simulink model "GS_model"  (R2018b)
settings: Solver=ode5  StartTime=0.0  StopTime=SimuStopTime  FixedStep=T_Simu  RelTol=1e-3
InitFcn:
  | Initial
undefined symbols (not defined in the file or in its folder): Aba10, Aba20, aeroCIP2006_S, aeroCIP2006_X, aeroCIP2006_Y, Agl0, Ass_kS, Ass_n1, Ass_n2, Ass_n3, Ass_n4, Ass_Noise, Ass_R, Ass_Resolution, Ass_TmOrder, AssA_Fix_Abs, AssB_Fix_Abs, AssC_Fix_Abs, AssD_Fix_Abs, AssE_Fix_Aps, AssF_Fix_Aps, C, c_max, c_min, Cd, CenterOfFigNX, CenterOfFigNY, CenterOfFigNZ, CenterOfFigP1, CenterOfFigP2, CenterOfFigPX, CenterOfFigPY, CenterOfFigPZ, Cmu, Crou, DEG2RAD, DiscIntNeverNeededParam, Eg_Dir, Eg_F, Eg_PrepareTime, Eg_r_L_L, Fw_Abf, Fw_Hmax, Fw_J, Fw_Spd0, Fw_Tmax, git_hash_BaseLine, git_hash_Project, Gnss_Noise_Pos, Gnss_Noise_Vel, Gnss_PropgationTime, GyroA_Fix_Abg, GyroA_Noise, GyroB_Fix_Abg, GyroB_Noise, GyroC_Fix_Abg, GyroC_Noise, GyroD_Fix_Abg, GyroD_Noise, h ... (+94)
libraries: simulink x308, sharedutil x46, aerolibutil x37, sharedtransform x31, vrlib x14, aerolibgravity2 x2
(part 3 of 20)

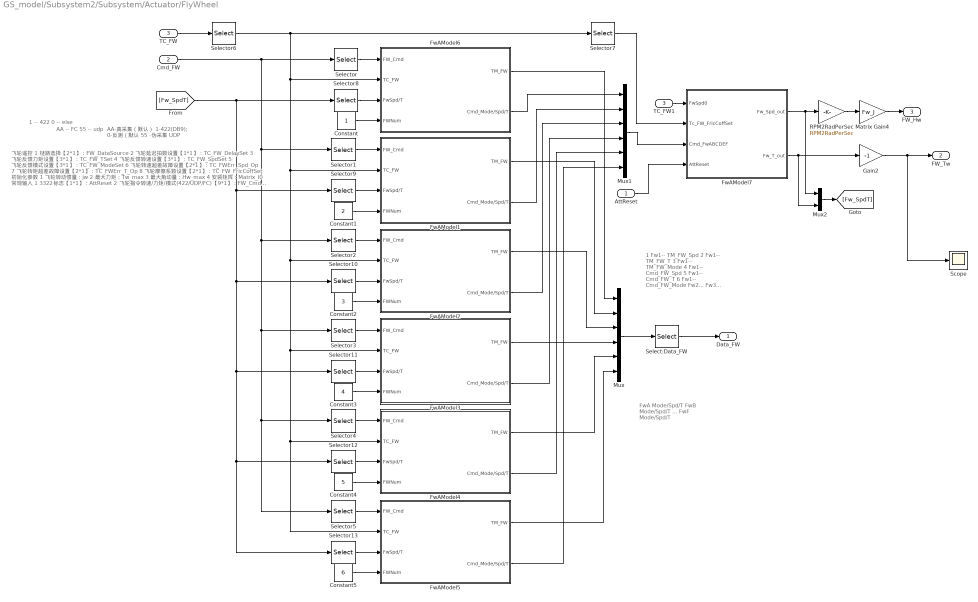
== system GS_model/Subsystem2/Subsystem/Actuator/FlyWheel ==
  note: FwA Mode/Spd/T
      | FwB Mode/Spd/T
      | ...
      | FwF Mode/Spd/T
  note: AA-真采集（默认）  1-422(DB9);
      |                                  0-反测（默认
      | 55 -伪采集                UDP
  note: 飞轮遥控
      | 1 链路选择【2*1】：FW_DataSource
      | 2 飞轮延迟拍数设置【1*1】：TC_FW_DelaySet
      | 3 飞轮反馈力矩设置【3*1】：TC_FW_TSet
      | 4 飞轮反馈转速设置【3*1】：TC_FW_SpdSet
      | 5 飞轮反馈模式设置【3*1】：TC_FW_ModeSet
      | 6 飞轮转速超差故障设置【2*1】：TC_FWErr_Spd_Op
      | 7 飞轮转矩超差故障设置【2*1】：TC_FWErr_T_Op
      | 8 飞轮摩擦系数设置【2*1】：TC_FW_FricCoffSet
      |
      | 初始化参数
      | 1 飞轮转动惯量：jw
      | 2 最大力矩：Tw_max
      | 3 最大角动量：Hw_max
      | 4 安装矩阵：Matrix_I0
      |
      | 常规输入
      | 1 3322标志【1*1】：AttReset
      | 2 飞轮指令转速/力矩/模式(422/UDP/FC)【9*1】：FW_Cmd
      |
      | 常规输出
      | 1 飞轮三轴力矩FW_Tw3
      | 2 飞轮三轴角动量：FW_Hw3
      |
      | 遥测输出
      | 1 飞轮反馈转速/力矩/模式【18*1】：Data_FW
  note: AA -- FC
      | 55 -- udp
  note: 1 -- 422
      | 0 -- else
  note: 1 Fw1-- TM_FW_Spd
      | 2 Fw1-- TM_FW_T
      | 3 Fw1-- TM_FW_Mode
      | 4 Fw1-- Cmd_FW_Spd
      | 5 Fw1-- Cmd_FW_T
      | 6 Fw1-- Cmd_FW_Mode
      |    Fw2...
      |    Fw3...
  AttReset : Inport
  Cmd_FW : Inport  Port=2
  TC_FW : Inport  Port=3
  Constant : Constant
  Constant1 : Constant  Value=2
  Constant2 : Constant  Value=3
  Constant3 : Constant  Value=4
  Constant4 : Constant  Value=5
  Constant5 : Constant  Value=6
  FwAModel1 : Subsystem
      mask Display: disp('FwAModel')
  FwAModel2 : Subsystem
      mask Display: disp('FwAModel')
  FwAModel3 : Subsystem
      mask Display: disp('FwAModel')
  FwAModel4 : Subsystem
      mask Display: disp('FwAModel')
  FwAModel5 : Subsystem
      mask Display: disp('FwAModel')
  FwAModel6 : Subsystem
      mask Display: disp('FwAModel')
  FwAModel7 : Subsystem
      mask Display: disp('FwModel')
  Gain2 : Gain  Gain=-1  SaturateOnIntegerOverflow=on  OutDataTypeStr=Inherit: Same as input  ParamDataTypeStr=Inherit: Same as input
  Matrix Gain4 : Gain  Gain=Fw_J  SaturateOnIntegerOverflow=on  OutDataTypeStr=Inherit: Same as input  ParamDataTypeStr=Inherit: Same as input
  Mux : Mux  Inputs=6
  Mux1 : Mux  Inputs=6
  Mux2 : Mux  Inputs=2
  RPM2RadPerSec : Gain  Gain=RPM2RadPerSec  SaturateOnIntegerOverflow=on  OutDataTypeStr=Inherit: Same as input  ParamDataTypeStr=Inherit: Same as input
  Scope : Scope
  Select:Data_FW : Selector  InputPortWidth=8*6  IndexOptions=Index vector (dialog)  Indices=[1:6 9:14 17:22 25:30 33:38 41:46]  OutputSizes=1
  Selector : Selector  InputPortWidth=18  IndexOptions=Index vector (dialog)  Indices=[1:3]  OutputSizes=1
  Selector1 : Selector  InputPortWidth=18  IndexOptions=Index vector (dialog)  Indices=[4:6]  OutputSizes=1
  Selector10 : Selector  InputPortWidth=12  IndexOptions=Index vector (dialog)  Indices=[3 9]  OutputSizes=1
  Selector11 : Selector  InputPortWidth=12  IndexOptions=Index vector (dialog)  Indices=[4 10]  OutputSizes=1
  Selector12 : Selector  InputPortWidth=12  IndexOptions=Index vector (dialog)  Indices=[5 11]  OutputSizes=1
  Selector13 : Selector  InputPortWidth=12  IndexOptions=Index vector (dialog)  Indices=[6 12]  OutputSizes=1
  Selector2 : Selector  InputPortWidth=18  IndexOptions=Index vector (dialog)  Indices=[7:9]  OutputSizes=1
  Selector3 : Selector  InputPortWidth=18  IndexOptions=Index vector (dialog)  Indices=[10:12]  OutputSizes=1
  Selector4 : Selector  InputPortWidth=18  IndexOptions=Index vector (dialog)  Indices=[13:15]  OutputSizes=1
  Selector5 : Selector  InputPortWidth=18  IndexOptions=Index vector (dialog)  Indices=[16:18]  OutputSizes=1
  Selector6 : Selector  InputPortWidth=23  IndexOptions=Index vector (dialog)  Indices=[3:17]  OutputSizes=1
  Selector7 : Selector  InputPortWidth=15  IndexOptions=Index vector (dialog)  Indices=15  OutputSizes=1
  Selector8 : Selector  InputPortWidth=12  IndexOptions=Index vector (dialog)  Indices=[1 7]  OutputSizes=1
  Selector9 : Selector  InputPortWidth=12  IndexOptions=Index vector (dialog)  Indices=[2 8]  OutputSizes=1
  TC_FW1 : InportShadow  Port=3
  Data_FW : Outport
  FW_Tw : Outport  Port=2
  FW_Hw : Outport  Port=3
  wires:
  Gain2/1 -> Scope/1, FW_Tw/1
  Matrix Gain4/1 -> FW_Hw/1
  Selector6/1 -> FwAModel5/2(TC_FW), FwAModel4/2(TC_FW), FwAModel3/2(TC_FW), FwAModel2/2(TC_FW), FwAModel1/2(TC_FW), FwAModel6/2(TC_FW), Selector7/1
  Selector5/1 -> FwAModel5/1(FW_Cmd)
  Selector4/1 -> FwAModel4/1(FW_Cmd)
  TC_FW/1 -> Selector6/1
  Cmd_FW/1 -> Selector5/1, Selector4/1, Selector3/1, Selector2/1, Selector1/1, Selector/1
  Select:Data_FW/1 -> Data_FW/1
  FwAModel7/1(Fw_Spd_out) -> Mux2/1, RPM2RadPerSec/1
  FwAModel5/1(TM_FW) -> Mux/6
  FwAModel4/1(TM_FW) -> Mux/5
  FwAModel3/1(TM_FW) -> Mux/4
  FwAModel2/1(TM_FW) -> Mux/3
  FwAModel1/1(TM_FW) -> Mux/2
  FwAModel6/1(TM_FW) -> Mux/1
  RPM2RadPerSec/1 -> Matrix Gain4/1
  FwAModel7/2(Fw_T_out) -> Mux2/2, Gain2/1
  Mux/1 -> Select:Data_FW/1
  Selector3/1 -> FwAModel3/1(FW_Cmd)
  Selector2/1 -> FwAModel2/1(FW_Cmd)
  Selector1/1 -> FwAModel1/1(FW_Cmd)
  Constant/1 -> FwAModel6/4(FWNum)
  Selector/1 -> FwAModel6/1(FW_Cmd)
  AttReset/1 -> FwAModel7/4(AttReset)
  Constant1/1 -> FwAModel1/4(FWNum)
  Constant2/1 -> FwAModel2/4(FWNum)
  Constant3/1 -> FwAModel3/4(FWNum)
  Constant4/1 -> FwAModel4/4(FWNum)
  Constant5/1 -> FwAModel5/4(FWNum)
  FwAModel6/2(Cmd_Mode/Spd/T) -> Mux1/1
  FwAModel1/2(Cmd_Mode/Spd/T) -> Mux1/2
  FwAModel2/2(Cmd_Mode/Spd/T) -> Mux1/3
  FwAModel3/2(Cmd_Mode/Spd/T) -> Mux1/4
  FwAModel4/2(Cmd_Mode/Spd/T) -> Mux1/5
  FwAModel5/2(Cmd_Mode/Spd/T) -> Mux1/6
  Selector7/1 -> FwAModel7/2(Tc_FW_FricCoffSet)
  Mux1/1 -> FwAModel7/3(Cmd_FwABCDEF)
  [Fw_SpdT] -> Selector8/1, Selector9/1, Selector10/1, Selector11/1, Selector12/1, Selector13/1
  Selector8/1 -> FwAModel6/3(FwSpd/T)
  Selector9/1 -> FwAModel1/3(FwSpd/T)
  Selector10/1 -> FwAModel2/3(FwSpd/T)
  Selector11/1 -> FwAModel3/3(FwSpd/T)
  Selector12/1 -> FwAModel4/3(FwSpd/T)
  Selector13/1 -> FwAModel5/3(FwSpd/T)
  Mux2/1 -> [Fw_SpdT]
  TC_FW1/1 -> FwAModel7/1(FwSpd0)

== system GS_model/Subsystem2/Subsystem/Actuator/Magnetorquer ==
  Tc_Mt : Inport
  Cmd_Mt : Inport  Port=2
  Mt_MathModel : Subsystem
  Mux : Mux  Inputs=2
  Data_Mt : Outport
  M_Mt : Outport  Port=2
  wires:
  Tc_Mt/1 -> Mt_MathModel/2(Tc_Mt)
  Cmd_Mt/1 -> Mt_MathModel/1(Cmd_Mt_Pro)
  Mt_MathModel/3(Tm_Mt) -> Mux/2
  Mt_MathModel/2(Cmd_Mt) -> Mux/1
  Mux/1 -> Data_Mt/1
  Mt_MathModel/1(M_Mt) -> M_Mt/1

== system GS_model/Subsystem2/Subsystem/Actuator/Motor ==
  Att_Reset : Inport
  Cmd_Motor : Inport  Port=2
  Tc_SADA : Inport  Port=3
  Tc_QV : Inport  Port=4
  UTC_1970 : Inport  Port=5
  Mux : Mux  Inputs=2
  QV : Subsystem
  Rate Transition{,1..2,4} (4 alike) : RateTransition  OutPortSampleTime=T_Simu
  SADA : Subsystem
  Selector1 : Selector  InputPortWidth=30  IndexOptions=Starting index (dialog)  Indices=1  OutputSizes=12
  Selector2 : Selector  InputPortWidth=30  IndexOptions=Starting index (dialog)  Indices=13  OutputSizes=8
  Selector3 : Selector  InputPortWidth=30  IndexOptions=Starting index (dialog)  Indices=21  OutputSizes=6
  Selector4 : Selector  InputPortWidth=30  IndexOptions=Starting index (dialog)  Indices=27  OutputSizes=4
  Motor_Agl/w/a : Outport
  Data_SADA : Outport  Port=2
  Data_QV : Outport  Port=3
  wires:
  Att_Reset/1 -> Rate Transition2/1
  Cmd_Motor/1 -> Selector3/1, Selector4/1, Selector2/1, Selector1/1
  Tc_SADA/1 -> Rate Transition/1
  SADA/1(Data_Motor_out) -> Data_SADA/1
  Rate Transition/1 -> SADA/1(TC_Motor_in)
  Rate Transition1/1 -> SADA/2(Cmd_Motor_in)
  Rate Transition2/1 -> QV/3(AttReset), SADA/3(AttReset)
  Selector1/1 -> Rate Transition1/1
  Selector2/1 -> QV/2(Cmd_Motor_in)
  Rate Transition4/1 -> QV/1(TC_Motor_in)
  Tc_QV/1 -> Rate Transition4/1
  QV/1(Data_Motor_out) -> Data_QV/1
  QV/2(SADA_Agl/w/a) -> Mux/2
  Selector4/1 -> QV/4(QVAgl_FC)
  Selector3/1 -> SADA/4(SADAAgl_FC)
  SADA/2(SADA_Agl/w/a) -> Mux/1
  Mux/1 -> Motor_Agl/w/a/1
  UTC_1970/1 -> QV/5(UTC_1970), SADA/5(UTC_1970)

== system GS_model/Subsystem2/Subsystem/PhysicsModel/DynModel ==
  note: % 输入：三轴外力（b系） 三轴外力矩（b系） 飞轮三轴角动量 飞轮三轴角动量微分
      | % 输入：a1角度/角速度/角加速度 p1角度/角速度/角加速度 附件1转序
      | % 输入：a2角度/角速度/角加速度 p2角度/角速度/角加速度 附件2转序
      | % 输入：上一拍微分方程输出值
      | % 输出：R(i系) Qib q   V(i系) wbi dq
  RV0 : Inport
  Orbit : Inport  Port=2
  Qio : Inport  Port=3
  Hw : Inport  Port=4
  Att0 : Inport  Port=5
  F(i) : Inport  Port=6
  Reset : Inport  Port=7
  AscDec : Inport  Port=8
  T(b) : Inport  Port=9
  Tc_MassPropertySet : Inport  Port=10
  Motor_Agl/w/a : Inport  Port=11
  AngularMomentumConservation : Subsystem
  Att：ECEF2VVLH : Subsystem
  Demux1 : Demux  Outputs=2
  Discrete Derivative : simulink/Discrete/Discrete Derivative  gainval=1.0  ICPrevScaledInput=0.0  OutMin=[]  OutMax=[]  OutDataType=fixdt(1, 16)  OutScaling=2^-10  DoSatur=off
  Display1 : Display
  EulerAngle_Inertial : Subsystem
  FlexDynModel : Subsystem
  Gain2 : Gain  Gain=RAD2DEG
  Hi : Scope  NumInputPorts=2
  Mux : Mux  Inputs=3
  Quaternion Norm : sharedutil/Quaternion Norm  aMode=aMode
      settings: SourceProductBaseCode=AE,PW,MT,VE,VP
  Quaternions to Rotation Angles : sharedtransform/Quaternions to Rotation Angles  rotationOrder=ZYX  aMode=aMode
      settings: SourceProductBaseCode=AE,PW,MT,VE,VP
  Scope : Scope
  Selector : Selector  InputPortWidth=3  IndexOptions=Index vector (dialog)  Indices=[3 2 1]  OutputSizes=1
  Selector2 : Selector  InputPortWidth=10  IndexOptions=Index vector (dialog)  Indices=[9]  OutputSizes=1
  Terminator : Terminator
  Terminator1 : Terminator
  Terminator2 : Terminator
  "wbi " : Scope
  Qib : Outport
  Qob : Outport  Port=2
  I : Outport  Port=3
  Cent : Outport  Port=4
  wbo : Outport  Port=5
  wbi : Outport  Port=6
  tag scope: Att_DLX=global, Euler_i=global, Euler_o=global, q_panel=global
  wires:
  Discrete Derivative/1 -> FlexDynModel/3(dHw_in)
  T(b)/1 -> FlexDynModel/4(T(b)_in)
  Att0/1 -> FlexDynModel/6(Att0_in)
  RV0/1 -> FlexDynModel/7(RV0_in)
  Motor_Agl/w/a/1 -> FlexDynModel/9(SADA_Agl/w/a_a/p_in)
  F(i)/1 -> FlexDynModel/8(F(i)_in)
  FlexDynModel/5(q_out) -> [q_panel]
  FlexDynModel/6(dq_out) -> Terminator2/1
  Orbit/1 -> Selector2/1
  Quaternions to Rotation Angles/1 -> Selector/1
  Demux1/1 -> EulerAngle_Inertial/1(Asc)
  EulerAngle_Inertial/1(EulerAngle_Inertial) -> [Euler_i]
  Demux1/2 -> EulerAngle_Inertial/2(Dec)
  AscDec/1 -> Demux1/1
  Gain2/1 -> "wbi "/1
  Reset/1 -> FlexDynModel/1(Reset_in)
  Hw/1 -> Discrete Derivative/1, AngularMomentumConservation/4(Hw_b), FlexDynModel/2(Hw_in)
  FlexDynModel/1(R_out) -> Terminator/1
  FlexDynModel/2(V_out) -> Terminator1/1
  AngularMomentumConservation/1(H_i) -> Hi/1
  [Spread] -> FlexDynModel/11(Spread_in)
  Selector2/1 -> Att：ECEF2VVLH/3(w00)
  Att：ECEF2VVLH/1(Qob) -> Qob/1, Quaternions to Rotation Angles/1
  Qio/1 -> FlexDynModel/5(Agl_Qio_in), Att：ECEF2VVLH/4(Qio)
  Tc_MassPropertySet/1 -> FlexDynModel/10(Tc_MassPropertySet_in)
  FlexDynModel/3(Agl_Qib_out) -> Att：ECEF2VVLH/1(Qib), AngularMomentumConservation/1(Qib), Quaternion Norm/1, EulerAngle_Inertial/3(Qib), Qib/1
  FlexDynModel/4(wbi_out) -> Att：ECEF2VVLH/2(wbi_b), AngularMomentumConservation/2(Wbi_b), Mux/3, Gain2/1, wbi/1
  FlexDynModel/7(I_out) -> AngularMomentumConservation/3(Ib), I/1
  FlexDynModel/8(Cent_out) -> Display1/1, Cent/1
  Selector/1 -> Mux/1, [Euler_o]
  Att：ECEF2VVLH/2(wbo_b) -> Mux/2, wbo/1
  Mux/1 -> [Att_DLX]
  Quaternion Norm/1 -> Scope/1
  AngularMomentumConservation/2(|H_i|) -> Hi/2

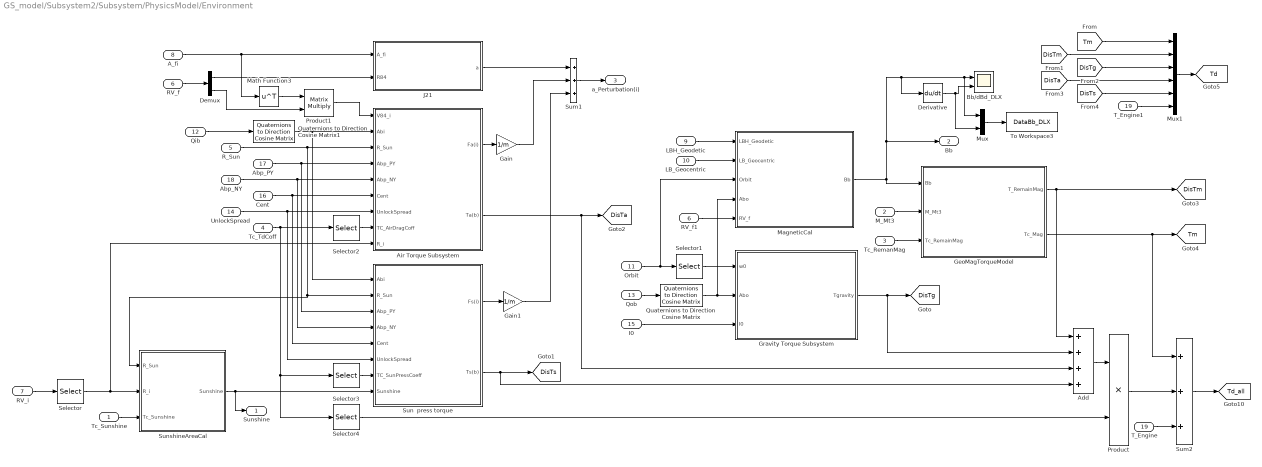
== system GS_model/Subsystem2/Subsystem/PhysicsModel/Environment ==
  Tc_Sunshine : Inport
  M_Mt3 : Inport  Port=2
  Tc_RemanMag : Inport  Port=3
  Tc_TdCoff : Inport  Port=4
  R_Sun : Inport  Port=5
  RV_f : Inport  Port=6
  RV_i : Inport  Port=7
  A_fi : Inport  Port=8
  LBH_Geodetic : Inport  Port=9
  LB_Geocentric : Inport  Port=10
  Orbit : Inport  Port=11
  Qib : Inport  Port=12
  Qob : Inport  Port=13
  UnlockSpread : Inport  Port=14
  I0 : Inport  Port=15
  Cent : Inport  Port=16
  Abp_PY : Inport  Port=17
  Abp_NY : Inport  Port=18
  T_Engine : Inport  Port=19
  Add : Sum  Inputs=++++
  Air Torque Subsystem : Subsystem
      mask Display: disp('AirDampModel')
  Bb/dBd_DLX : Scope  NumInputPorts=2
  Demux : Demux  Outputs=[3;3]
  Derivative : Derivative
  Gain : Gain  Gain=1/m
  Gain1 : Gain  Gain=1/m
  GeoMagTorqueModel : Subsystem
      mask Display: disp('GeoMagTorqueModel')
  Gravity Torque Subsystem : Subsystem
      mask Display: disp('GravityTorque')
  J21 : Subsystem
  MagneticCal : Subsystem
  Math Function3 : Math  Operator=transpose  SaturateOnIntegerOverflow=on
  Mux : Mux  Inputs=2
  Mux1 : Mux  Inputs=6
  Product : Product
  Product1 : Product  Multiplication=Matrix(*)
  Quaternions to Direction Cosine Matrix : sharedtransform/Quaternions to  Direction Cosine Matrix  aMode=aMode
      settings: SourceProductBaseCode=AE,PW,MT,VE,VP
  Quaternions to Direction Cosine Matrix1 : sharedtransform/Quaternions to  Direction Cosine Matrix  aMode=aMode
      settings: SourceProductBaseCode=AE,PW,MT,VE,VP
  RV_f1 : InportShadow  Port=6
  Selector : Selector  InputPortWidth=6  IndexOptions=Index vector (dialog)  Indices=[1 2 3]  OutputSizes=1
  Selector1 : Selector  InputPortWidth=10  IndexOptions=Index vector (dialog)  Indices=9  OutputSizes=1
  Selector2 : Selector  InputPortWidth=3  IndexOptions=Index vector (dialog)  Indices=1  OutputSizes=1
  Selector3 : Selector  InputPortWidth=3  IndexOptions=Index vector (dialog)  Indices=2  OutputSizes=1
  Selector4 : Selector  InputPortWidth=3  IndexOptions=Index vector (dialog)  Indices=3  OutputSizes=1
  Sum1 : Sum  Inputs=+++
  Sum2 : Sum  Inputs=3
  Sun  press torque : Subsystem
      mask Display: disp('SunPressModel')
  SunshineAreaCal : Subsystem
  T_Engine1 : InportShadow  Port=19
  To Workspace3 : ToWorkspace  VariableName=DataBb_DLX  SampleTime=-1
  Sunshine : Outport
  Bb : Outport  Port=2
  a_Perturbation(i) : Outport  Port=3
  tag scope: DisTa=global, DisTg=global, DisTm=global, DisTs=global, Td=global, Td_all=global, Tm=global
  wires:
  RV_f/1 -> Demux/1
  Demux/1 -> J21/2(R84)
  Math Function3/1 -> Product1/1
  A_fi/1 -> Math Function3/1, J21/1(A_fi)
  M_Mt3/1 -> GeoMagTorqueModel/2(M_Mt3)
  Demux/2 -> Product1/2
  Product1/1 -> Air Torque Subsystem/1(V84_i)
  Qib/1 -> Quaternions to Direction Cosine Matrix1/1
  R_Sun/1 -> SunshineAreaCal/1(R_Sun), Sun  press torque/2(R_Sun), Air Torque Subsystem/3(R_Sun)
  Abp_PY/1 -> Sun  press torque/3(Abp_PY), Air Torque Subsystem/4(Abp_PY)
  Abp_NY/1 -> Sun  press torque/4(Abp_NY), Air Torque Subsystem/5(Abp_NY)
  Cent/1 -> Sun  press torque/5(Cent), Air Torque Subsystem/6(Cent)
  UnlockSpread/1 -> Sun  press torque/6(UnlockSpread), Air Torque Subsystem/7(UnlockSpread)
  Tc_TdCoff/1 -> Selector4/1, Selector3/1, Selector2/1
  RV_i/1 -> Selector/1
  Selector/1 -> SunshineAreaCal/2(R_i), Air Torque Subsystem/9(R_i)
  Sum1/1 -> a_Perturbation(i)/1
  Air Torque Subsystem/1(Fa(i)) -> Gain/1
  I0/1 -> Gravity Torque Subsystem/3(I0)
  Qob/1 -> Quaternions to Direction Cosine Matrix/1
  Selector1/1 -> Gravity Torque Subsystem/1(w0)
  Orbit/1 -> Selector1/1, MagneticCal/3(Orbit)
  Quaternions to Direction Cosine Matrix/1 -> MagneticCal/4(Abo), Gravity Torque Subsystem/2(Abo)
  Selector2/1 -> Air Torque Subsystem/8(TC_AirDragCoff)
  Selector3/1 -> Sun  press torque/7(TC_SunPressCoeff)
  SunshineAreaCal/1(Sunshine) -> Sun  press torque/8(Sunshine), Sunshine/1
  Sun  press torque/1(Fs(i)) -> Gain1/1
  Gain1/1 -> Sum1/3
  LB_Geocentric/1 -> MagneticCal/2(LB_Geocentric)
  LBH_Geodetic/1 -> MagneticCal/1(LBH_Geodetic)
  MagneticCal/1(Bb) -> GeoMagTorqueModel/1(Bb), Derivative/1, Mux/1, Bb/dBd_DLX/1, Bb/1
  Tc_RemanMag/1 -> GeoMagTorqueModel/3(Tc_RemainMag)
  Gravity Torque Subsystem/1(Tgravity) -> Add/2, [DisTg]
  GeoMagTorqueModel/2(Tc_Mag) -> Sum2/1, [Tm]
  Quaternions to Direction Cosine Matrix1/1 -> Sun  press torque/1(Abi), Air Torque Subsystem/2(Abi)
  Sum2/1 -> [Td_all]
  Tc_Sunshine/1 -> SunshineAreaCal/3(Tc_Sunshine)
  Sun  press torque/2(Ts(b)) -> [DisTs], Add/4
  Air Torque Subsystem/2(Ta(b)) -> Add/3, [DisTa]
  GeoMagTorqueModel/1(T_RemainMag) -> Add/1, [DisTm]
  J21/1(a) -> Sum1/1
  Gain/1 -> Sum1/2
  Derivative/1 -> Mux/2, Bb/dBd_DLX/2
  Mux/1 -> To Workspace3/1
  Add/1 -> Product/1
  Selector4/1 -> Product/2
  Product/1 -> Sum2/2
  T_Engine/1 -> Sum2/3
  Mux1/1 -> [Td]
  [DisTm] -> Mux1/2
  [Tm] -> Mux1/1
  [DisTg] -> Mux1/3
  [DisTa] -> Mux1/4
  [DisTs] -> Mux1/5
  T_Engine1/1 -> Mux1/6
  RV_f1/1 -> MagneticCal/5(RV_f)

== system GS_model/Subsystem2/Subsystem/PhysicsModel/Environment1 ==
  JDC_2000 : Inport
  Constant : Constant  Value=[0;0;0]
  Constant1 : Constant  Value=[0;0]
  MATLAB Function : MATLAB Function  TreatAsAtomicUnit=on
  AscDec_Sun : Outport
  R_Moon : Outport  Port=2
  AscDec_Moon : Outport  Port=3
  R_Sun : Outport  Port=4
  wires:
  JDC_2000/1 -> MATLAB Function/1(JDC_2000)
  MATLAB Function/2(AscDec_Sun) -> AscDec_Sun/1
  Constant/1 -> R_Moon/1
  Constant1/1 -> AscDec_Moon/1
  MATLAB Function/1(R_Sun) -> R_Sun/1

== system GS_model/Subsystem2/Subsystem/PhysicsModel/Orbit ==
  UTC_1970 : Inport
  Tc_Reset : Inport  Port=2
  Tc_Orbit : Inport  Port=3
  F_Engine(b) : Inport  Port=4
  Qib : Inport  Port=5
  a_Perturbation : Inport  Port=6
  Compute osculating elements : Subsystem
  Engine : Subsystem
  Fcn : Fcn  Expr=u(5)+u(6)
  Gain : Gain  Gain=180/pi
  MATLAB Function : MATLAB Function  TreatAsAtomicUnit=on
  MATLAB Function1 : MATLAB Function  TreatAsAtomicUnit=on
  Mux : Mux  Inputs=2
  Mux1 : Mux  Inputs=2
  Mux2 : Mux  Inputs=3
  Mux3 : Mux  Inputs=3
  Qob 2 Qib : Subsystem
  RV_i2RV_f : Subsystem
  Selector : Selector  InputPortWidth=2  IndexOptions=Index vector (dialog)  Indices=1  OutputSizes=1
  Subsystem : Subsystem
  Subsystem1 : Subsystem
  u : Scope
  RV_f : Outport
  RV_i : Outport  Port=2
  Afi : Outport  Port=3
  LBH_Geodetic : Outport  Port=4
  LBH_Geocentic : Outport  Port=5
  Orbit : Outport  Port=6
  Qio : Outport  Port=7
  RV0 : Outport  Port=8
  tag scope: LBH=global, Orbit=global
  wires:
  a_Perturbation/1 -> Subsystem/3(a_Perturbation)
  Subsystem/2(V_i) -> RV_i2RV_f/2(V_i), Mux/2, Compute osculating elements/2(v_xyz)
  Subsystem/1(R_i) -> RV_i2RV_f/1(R_i), Mux/1, Compute osculating elements/1(r_xyz)  "不对"
  Mux/1 -> RV_i/1
  Compute osculating elements/1(OrbitElement) -> Fcn/1, [Orbit], Qob 2 Qib/1(OrbitElement), Orbit/1
  UTC_1970/1 -> Subsystem1/1(UTC_1970)
  RV_i2RV_f/1(R_f) -> Mux1/1, MATLAB Function/1(R_84)
  Subsystem1/1(Afi) -> Afi/1, RV_i2RV_f/3(Afi)
  RV_i2RV_f/2(V_f) -> Mux1/2
  Mux1/1 -> RV_f/1
  MATLAB Function/1(L_Geodetic) -> Mux2/1
  MATLAB Function/2(B_Geodetic) -> Mux2/2
  MATLAB Function/3(H_Geodetic) -> Mux2/3
  MATLAB Function/4(L_Geocentric) -> Mux3/1
  MATLAB Function/5(B_Geocentric) -> Mux3/2
  Selector/1 -> Subsystem/1(Tc_Orbit_Reset)
  Tc_Reset/1 -> Selector/1
  Qob 2 Qib/1(Qio) -> Qio/1
  Tc_Orbit/1 -> MATLAB Function1/1(Orbit)
  MATLAB Function1/1(RV_i) -> RV0/1, Subsystem/2(RV0)
  Mux2/1 -> LBH_Geodetic/1, [LBH]  "地理"
  Mux3/1 -> LBH_Geocentic/1  "地心"
  Fcn/1 -> Gain/1
  Gain/1 -> u/1
  Qib/1 -> Engine/2(Qib)
  F_Engine(b)/1 -> Engine/1(F_Engine(b))
  Engine/1(F_Engine(i)) -> Subsystem/4(F_EP)
  MATLAB Function/6(H_Geocentric) -> Mux3/3

== system GS_model/Subsystem2/Subsystem/PhysicsModel/Subsystem3 ==
  M_Mt : Inport
  H_Fw : Inport  Port=2
  T_Fw : Inport  Port=3
  Agl/w/a_SADA : Inport  Port=4
  Gain : Gain  Gain=Mt_Abm  Multiplication=Matrix(K*u)
  Gain1 : Gain  Gain=Fw_Abf  Multiplication=Matrix(K*u)
  Gain2 : Gain  Gain=Fw_Abf  Multiplication=Matrix(K*u)
  Selector1 : Selector  InputPortWidth=30  IndexOptions=Index vector (dialog)  Indices=1:12  OutputSizes=1
  Subsystem1 : Subsystem
  Terminator : Terminator
  Terminator1 : Terminator
  Abp_PY : Outport
  Abp_NY : Outport  Port=2
  M_Dyn : Outport  Port=3
  H_Dyn : Outport  Port=4
  tag scope: T_Fw3=global
  wires:
  Gain2/1 -> H_Dyn/1
  Gain/1 -> M_Dyn/1
  M_Mt/1 -> Gain/1
  T_Fw/1 -> Gain1/1
  H_Fw/1 -> Gain2/1
  Gain1/1 -> [T_Fw3]
  Subsystem1/1(Abp1) -> Abp_PY/1
  Subsystem1/2(Aba1) -> Terminator/1
  Subsystem1/3(Abp2) -> Abp_NY/1
  Subsystem1/4(Aba2) -> Terminator1/1
  Agl/w/a_SADA/1 -> Selector1/1
  Selector1/1 -> Subsystem1/1(Agl/w/a_SADA)

== system GS_model/Subsystem2/Subsystem/PhysicsModel/Time ==
  UTC0_1970 : Inport
  Reset : Inport  Port=2
  Clock : Clock
  Constant : Constant  Value=UTC_1970to2000
  Constant2 : Constant  Value=T_LeapSec
  Gain : Gain  Gain=1/K_Day2Sec
  Gain1 : Gain  Gain=1/K_Century2Day
  Selector : Selector  InputPortWidth=2  IndexOptions=Index vector (dialog)  Indices=1  OutputSizes=1
  Subsystem : Subsystem
  Sum : Sum  Inputs=|+-
  Sum1 : Sum  Inputs=|++
  Sum2 : Sum  Inputs=-+|
  Sum3 : Sum  Inputs=|++
  JDC_2000 : Outport
  TAI_1970 : Outport  Port=2
  UTC_1970 : Outport  Port=3
  wires:
  Sum/1 -> Gain/1
  Constant/1 -> Sum/2
  Gain/1 -> Gain1/1
  Gain1/1 -> JDC_2000/1
  UTC0_1970/1 -> Sum3/2
  Reset/1 -> Selector/1
  Constant2/1 -> Sum1/1
  Sum3/1 -> Sum1/2, UTC_1970/1, Sum/1
  Sum1/1 -> TAI_1970/1
  Selector/1 -> Subsystem/Trigger
  Clock/1 -> Sum2/2, Subsystem/1(In1)
  Subsystem/1(Out1) -> Sum2/1
  Sum2/1 -> Sum3/1

== system GS_model/Subsystem2/Subsystem/Sensor/Ass ==
  note: 太敏遥控
      | 1 电池片设置【6*1】：TC_AssGNDSet
      | 2 不变故障【2*1】：TC_AssErr_Constant
      | 3 野值故障【2*1】：TC_AssErr_WildValue
      | 4 跳变故障【4*1】：TC_AssErr_Jump
      | 5 波动故障【3*1】：TC_AssErr_Wave
      |
      | 初始化参数
      | 1 安装矩阵【3*3】：AssA/B/C/D_Fix_Abs (Body)
      | 2 安装矩阵【3*3】：AssE_Fix_Aps (PY)
      | 3 安装矩阵【3*3】：AssF_Fix_Aps (NY)
      | 4 太敏电阻【1*1】：R_Ass
      |
      | 常规输入
      | 1 光照标志【1*1】：Sunshine
      | 2 本体系太阳矢量【3*1】：Sun_b
      | 3 正Y帆板转移矩阵【3*3】：Abp_PY
      | 4 负Y帆板转移矩阵【3*3】：Abp_NY
      |
      | 输出
      | 1 太敏电池片电流【24*1】：Data_Ass
  Sun_b : Inport
  Sunshine : Inport  Port=2
  TC_Ass : Inport  Port=3
  Abp_PY : Inport  Port=4
  Abp_NY : Inport  Port=5
  BodyAss(A&B&C&D)Model : Subsystem
      mask Display: disp('BodyAss(A&B&C&D)Model')
  Mux : Mux  Inputs=2
  SolarPanelAss(E&F)Model : Subsystem
      mask Display: disp('SolarPanelAss(E&F)Model');
  Data_Ass : Outport
  wires:
  Sunshine/1 -> SolarPanelAss(E&F)Model/1(Sunshine), BodyAss(A&B&C&D)Model/1(Sunshine)
  Sun_b/1 -> SolarPanelAss(E&F)Model/2(Sun_b), BodyAss(A&B&C&D)Model/2(Sun_b)
  TC_Ass/1 -> SolarPanelAss(E&F)Model/3(TC_Ass), BodyAss(A&B&C&D)Model/3(TC_Ass)
  BodyAss(A&B&C&D)Model/1(TM_Data_AssA&B&C&D) -> Mux/1
  Abp_PY/1 -> SolarPanelAss(E&F)Model/4(Abp_PY)
  Abp_NY/1 -> SolarPanelAss(E&F)Model/5(Abp_NY)
  SolarPanelAss(E&F)Model/1(TM_Data_AssE&F) -> Mux/2
  Mux/1 -> Data_Ass/1

== system GS_model/Subsystem2/Subsystem/Sensor/GNSS ==
  note: GNSS遥控
      | 1 位置设置【4*1】：TC_GNSS_GNDSet_Pos
      | 2 速度设置【4*1】：TC_GNSS_GNDSet_Spd
      | 3 位置不变故障【1*1】：TC_GNSSErr_PosConstant
      | 4 速度不变故障【1*1】：TC_GNSSErr_SpdConstant
      | 5 位置野值故障【1*1】：TC_GNSSErr_PosWildValue
      | 6 速度野值故障【1*1】：TC_GNSSErr_SpdWildValue
      | 7 外推时间【1*1】：TC_GNSS_T
      |
      | 初始化参数
      | 无
      |
      | 常规输入
      | 1 UTC1970【1*1】
      | 2 JDC2000【1*1】
      | 3 RV_J2000【6*1】
      |
      | 输出
      | GNSS时间/位置/速度/定位位置/定位速度【13*1】
  RV_f : Inport
  TC_GNSS : Inport  Port=2
  TAI1970 : Inport  Port=3
  UTC_1970 : Inport  Port=4
  Demux : Demux  Outputs=[3;3]
  Demux1 : Demux  Outputs=2
  Enabled Subsystem : Subsystem  TreatAsAtomicUnit=on
  GNSSErrModel : Subsystem
      mask Display: disp('GNSSErrModel')
  GNSS_IntegerSecond_Judge : Subsystem
  Gnss_Noise_Pos : RandomNumber  Mean=[0;0;0]  Variance=(Gnss_Noise_Pos/3).^2  Seed=[1;2;3]  SampleTime=T_Simu
  Gnss_Noise_Vel : RandomNumber  Mean=[0;0;0]  Variance=(Gnss_Noise_Vel/3).^2  Seed=[4;5;6]  SampleTime=T_Simu
  Mux : Mux  Inputs=5
  Mux1 : Mux  Inputs=2
  Mux2 : Mux  Inputs=2
  Mux3 : Mux  Inputs=2
  Orbit : Subsystem
      mask Display: disp('GNSS Propagation')
  Orbit1 : Subsystem
      mask Display: disp('GNSS Propagation')
  Sum : Sum  Inputs=|++
  Sum1 : Sum  Inputs=|++
  Sum2 : Sum  Inputs=|++
  Data_GNSS : Outport
  wires:
  Demux/1 -> GNSSErrModel/2(R_84)
  Demux/2 -> GNSSErrModel/3(V_84)
  GNSS_IntegerSecond_Judge/1(Boolean) -> Enabled Subsystem/Trigger
  TAI1970/1 -> Mux/1, GNSS_IntegerSecond_Judge/1(TAI1970)
  GNSSErrModel/1(TM_R_84) -> Mux/2
  GNSSErrModel/2(TM_V_84) -> Mux/3
  Mux/1 -> Enabled Subsystem/1(In1)
  Enabled Subsystem/1(Out1) -> Data_GNSS/1
  UTC_1970/1 -> Orbit1/2(UTC_1970), Orbit/2(UTC_1970)
  TC_GNSS/1 -> GNSSErrModel/1(TC_GNSS)
  Gnss_Noise_Vel/1 -> Mux1/2
  Gnss_Noise_Pos/1 -> Mux1/1
  RV_f/1 -> Sum/1
  Sum/1 -> Demux/1
  Demux1/1 -> Orbit/1("\tTC_GNSS_PropagationTime")
  Demux1/2 -> Orbit1/1("\tTC_GNSS_PropagationTime")
  Orbit1/1(R_f) -> Mux3/1
  Orbit1/2(V_f) -> Mux3/2
  Orbit/1(R_f) -> Mux2/1
  Orbit/2(V_f) -> Mux2/2
  Mux2/1 -> Sum1/1
  Mux3/1 -> Sum2/1
  Sum1/1 -> Mux/4
  Sum2/1 -> Mux/5
  GNSSErrModel/3(TC_GNSS_PropagationTime) -> Demux1/1
  Mux1/1 -> Sum1/2, Sum2/2, Sum/2

== system GS_model/Subsystem2/Subsystem/Sensor/Gyro ==
  note: 陀螺遥控
      | 1 TC_GyroGNDSet
      | 2 TC_GyroErr_Constant
      | 3 TC_GyroErr_WildValue
      | 4 TC_GyroErr_Jump
      | 5 TC_GyroErr_Wave
      | 6 TC_GyroDriftSet
      |
      | 初始化参数
      | 1   GyroA_Fix
      | 2   GyroB_Fix
      | 3   GyroC_Fix
      | 4   GyroD_Fix
      | 5   GyroA_Drift
      | 6   GyroB_Drift
      | 7   GyroC_Drift
      | 8   GyroD_Drift
      | 9   GyroA_Noise
      | 10 GyroB_Noise
      | 11 GyroC_Noise
      | 12 GyroD_Noise
      |
      | 常规输入
      | 1 Wbi
      |
      |
      | 输出
      | 1 Wgi_GyroA
      | 2 Wgi_GyroB
      | 3 Wgi_GyroC
      | 4 Wgi_GyroD
  Wbi_b : Inport
  Tc_Gyro : Inport  Port=2
  Constant : Constant
  Constant1 : Constant  Value=GyroA_Fix_Abg
  Constant10 : Constant  Value=GyroD_Fix_Abg
  Constant3 : Constant  Value=2
  Constant4 : Constant  Value=GyroB_Fix_Abg
  Constant6 : Constant  Value=3
  Constant7 : Constant  Value=GyroC_Fix_Abg
  Constant9 : Constant  Value=4
  GyroAModel : Subsystem
  GyroA_Noise : RandomNumber  Mean=[0;0;0]  Variance=(GyroA_Noise/180*pi/3).^2  Seed=[1;2;3]  SampleTime=T_Simu
  GyroBModel : Subsystem
  GyroB_Noise : RandomNumber  Mean=[0;0;0]  Variance=(GyroB_Noise/180*pi/3).^2  Seed=[1;2;3]+3  SampleTime=T_Simu
  GyroCModel : Subsystem
  GyroC_Noise : RandomNumber  Mean=[0;0;0]  Variance=(GyroC_Noise/180*pi/3).^2  Seed=[1;2;3]+6  SampleTime=T_Simu
  GyroDModel : Subsystem
  GyroD_Noise : RandomNumber  Mean=[0;0;0]  Variance=(GyroD_Noise/180*pi/3).^2  Seed=[1;2;3]+9  SampleTime=T_Simu
  Mux : Mux
  Data_Gyro : Outport
  wires:
  Wbi_b/1 -> GyroCModel/1(Wbi_b), GyroDModel/1(Wbi_b), GyroBModel/1(Wbi_b), GyroAModel/1(Wbi_b)
  Tc_Gyro/1 -> GyroAModel/4(TC_Gyro), GyroDModel/4(TC_Gyro), GyroCModel/4(TC_Gyro), GyroBModel/4(TC_Gyro)
  Constant1/1 -> GyroAModel/2(Gyro_Fix_Abg)
  GyroA_Noise/1 -> GyroAModel/3(Gyro_Noise)
  Mux/1 -> Data_Gyro/1
  GyroAModel/1(TM_Gyro_Wgi) -> Mux/1
  Constant/1 -> GyroAModel/5(Gyro_Num)
  GyroBModel/1(TM_Gyro_Wgi) -> Mux/2
  GyroCModel/1(TM_Gyro_Wgi) -> Mux/3
  GyroDModel/1(TM_Gyro_Wgi) -> Mux/4
  Constant4/1 -> GyroBModel/2(Gyro_Fix_Abg)
  GyroB_Noise/1 -> GyroBModel/3(Gyro_Noise)
  Constant3/1 -> GyroBModel/5(Gyro_Num)
  Constant7/1 -> GyroCModel/2(Gyro_Fix_Abg)
  GyroC_Noise/1 -> GyroCModel/3(Gyro_Noise)
  Constant6/1 -> GyroCModel/5(Gyro_Num)
  Constant10/1 -> GyroDModel/2(Gyro_Fix_Abg)
  GyroD_Noise/1 -> GyroDModel/3(Gyro_Noise)
  Constant9/1 -> GyroDModel/5(Gyro_Num)

== system GS_model/Subsystem2/Subsystem/Sensor/Magnetometer ==
  note: 磁强计遥控
      | 1 TC_MmGNDSet
      | 2 TC_MmErr_Constant
      | 3 TC_MmErr_WildValue
      | 4 TC_MmErr_Jump
      | 5 TC_MmErr_Wave
      |
      | 初始化参数
      | 1   MmA_Fix_Abm
      | 2   MmB_Fix_Abm
      | 3   MmC_Fix_Abm
      | 4   MmD_Fix_Abm
      | 5   MmA_MtInflunce_Coff
      | 6   MmB_MtInflunce_Coff
      | 7   MmC_MtInflunce_Coff
      | 8   MmD_MtInflunce_Coff
      | 9   Mt_MaxCurrent_Coff
      | 10 MmA_Noise
      | 11 MmB_Noise
      | 12 MmC_Noise
      | 13 MmD_Noise
      |
      | 常规输入
      | 1 Bb
      | 2 M_Mt
      |
      |
      | 输出
      | 1 MmA_MagneticIntensity
      | 2 MmB_MagneticIntensity
      | 3 MmC_MagneticIntensity
      | 4 MmD_MagneticIntensity
  Bb : Inport
  M_Mt : Inport  Port=2
  Tc_Mm : Inport  Port=3
  Constant11 : Constant  Value=MmB_Fix_Abm
  Constant12 : Constant  Value=MmB_MtInflunce_Coff
  Constant13 : Constant  Value=2
  Constant14 : Constant  Value=MmC_Fix_Abm
  Constant15 : Constant  Value=MmC_MtInflunce_Coff
  Constant16 : Constant  Value=3
  Constant17 : Constant  Value=MmD_Fix_Abm
  Constant18 : Constant  Value=MmD_MtInflunce_Coff
  Constant19 : Constant  Value=4
  Constant2 : Constant  Value=MmA_Fix_Abm
  Constant5 : Constant  Value=MmA_MtInflunce_Coff
  Constant8 : Constant
  Gain : Gain
  MmA_Noise : RandomNumber  Mean=[0;0;0]  Variance=(MmA_Noise/3).^2  Seed=[1;2;3]  SampleTime=T_Simu
  MmB_Noise : RandomNumber  Mean=[0;0;0]  Variance=(MmB_Noise/3).^2  Seed=[1;2;3]+3  SampleTime=T_Simu
  MmC_Noise : RandomNumber  Mean=[0;0;0]  Variance=(MmC_Noise/3).^2  Seed=[1;2;3]+6  SampleTime=T_Simu
  MmD_Noise : RandomNumber  Mean=[0;0;0]  Variance=(MmD_Noise/3).^2  Seed=[1;2;3]+9  SampleTime=T_Simu
  MmModel1 : Subsystem
  MmModel2 : Subsystem
  MmModel3 : Subsystem
  MmModel4 : Subsystem
  Mux1 : Mux
  Data_Mm : Outport
  wires:
  Constant2/1 -> MmModel1/3(Mm_Fix_Abm)
  Constant5/1 -> MmModel1/4(Mm_MtInflunce_Coff)
  MmA_Noise/1 -> MmModel1/5(Mm_Noise)
  Constant8/1 -> MmModel1/7(Mm_Num)
  Constant11/1 -> MmModel2/3(Mm_Fix_Abm)
  Constant12/1 -> MmModel2/4(Mm_MtInflunce_Coff)
  Constant13/1 -> MmModel2/7(Mm_Num)
  MmB_Noise/1 -> MmModel2/5(Mm_Noise)
  Constant14/1 -> MmModel3/3(Mm_Fix_Abm)
  Constant15/1 -> MmModel3/4(Mm_MtInflunce_Coff)
  Constant16/1 -> MmModel3/7(Mm_Num)
  MmC_Noise/1 -> MmModel3/5(Mm_Noise)
  Constant17/1 -> MmModel4/3(Mm_Fix_Abm)
  Constant18/1 -> MmModel4/4(Mm_MtInflunce_Coff)
  Tc_Mm/1 -> MmModel2/6(TC_Mm), MmModel4/6(TC_Mm), MmModel3/6(TC_Mm), MmModel1/6(TC_Mm)
  Constant19/1 -> MmModel4/7(Mm_Num)
  MmD_Noise/1 -> MmModel4/5(Mm_Noise)
  MmModel1/1(TM_Mm) -> Mux1/1
  MmModel2/1(TM_Mm) -> Mux1/2
  MmModel3/1(TM_Mm) -> Mux1/3
  MmModel4/1(TM_Mm) -> Mux1/4
  Mux1/1 -> Data_Mm/1
  M_Mt/1 -> MmModel2/2(M_Mt), MmModel4/2(M_Mt), MmModel3/2(M_Mt), MmModel1/2(M_Mt)
  Bb/1 -> Gain/1
  Gain/1 -> MmModel2/1(Bb), MmModel4/1(Bb), MmModel3/1(Bb), MmModel1/1(Bb)

== system GS_model/Subsystem2/Subsystem/Sensor/StA&B&C&DModel1 ==
  note: 星敏遥控
      | 1 TC_StFixErr
      | 2 TC_StNoiseCoff
      | 3 TC_StGNDSet
      | 4 TC_StErr_Constant
      | 5 TC_StErr_WildValue
      | 6 TC_StErr_Jump
      | 7 TC_StErr_Wave
      |
      | 初始化参数
      | 1 Qbs_StAFix
      | 2 Qbs_StBFix
      | 3 Qbs_StCFix
      | 4 Qbs_StDFix
      | 5 StANoise
      | 6 StBNoise
      | 7 StCNoise
      | 8 StDNoise
      |
      | 常规输入
      | 1 Qib
      | 2 UTC_1970
      |
      | 输出
      | 1 StA_Time/Qis_StA/W_StA
      | 2 StB_Time/Qis_StB/W_StB
      | 3 StC_Time/Qis_StC/W_StC
      | 4 StD_Time/Qis_StD/W_StD
  Qib : Inport
  Sun_b : Inport  Port=2
  Sunshine : Inport  Port=3
  TC_St : Inport  Port=4
  UTC_1970 : Inport  Port=5
  Qob : Inport  Port=6
  Constant : Constant  Value=StA_Fix_Qsb
  Constant1 : Constant
  Constant10 : Constant  Value=StC_Fix_Qsb
  Constant11 : Constant  Value=StD_Fix_Qsb
  Constant2 : Constant  Value=2
  Constant3 : Constant  Value=3
  Constant4 : Constant  Value=4
  Constant5 : Constant  Value=St_SEA
  Constant6 : Constant  Value=St_EEA
  Constant9 : Constant  Value=StB_Fix_Qsb
  Mux : Mux  Inputs=8
  Mux1 : Mux  Inputs=2
  Selector1 : Selector  InputPortWidth=4  IndexOptions=Index vector (dialog)  Indices=1  OutputSizes=1
  Selector2 : Selector  InputPortWidth=4  IndexOptions=Index vector (dialog)  Indices=1  OutputSizes=1
  Selector3 : Selector  InputPortWidth=4  IndexOptions=Index vector (dialog)  Indices=2  OutputSizes=1
  Selector4 : Selector  InputPortWidth=4  IndexOptions=Index vector (dialog)  Indices=2  OutputSizes=1
  Selector5 : Selector  InputPortWidth=4  IndexOptions=Index vector (dialog)  Indices=3  OutputSizes=1
  Selector6 : Selector  InputPortWidth=4  IndexOptions=Index vector (dialog)  Indices=3  OutputSizes=1
  Selector7 : Selector  InputPortWidth=4  IndexOptions=Index vector (dialog)  Indices=4  OutputSizes=1
  Selector8 : Selector  InputPortWidth=4  IndexOptions=Index vector (dialog)  Indices=4  OutputSizes=1
  StAMathModel : Subsystem
      mask Display: disp('StAModel');
  StAMathModel1 : Subsystem
      mask Display: disp('StAModel');
  StAMathModel2 : Subsystem
      mask Display: disp('StAModel');
  StAMathModel3 : Subsystem
      mask Display: disp('StAModel');
  StANoise : RandomNumber  Mean=[0;0;0]  Variance=(StANoise*pi/180/3600/3).^2  Seed=[1;2;3]  SampleTime=T_Simu
  StBNoise : RandomNumber  Mean=[0;0;0]  Variance=(StBNoise*pi/180/3600/3).^2  Seed=[4;5;6]  SampleTime=T_Simu
  StCNoise : RandomNumber  Mean=[0;0;0]  Variance=(StCNoise*pi/180/3600/3).^2  Seed=[7;8;9]  SampleTime=T_Simu
  StDNoise : RandomNumber  Mean=[0;0;0]  Variance=(StDNoise*pi/180/3600/3).^2  Seed=[10;11;12]  SampleTime=T_Simu
  Subsystem : Subsystem
      mask Display: disp('StTimeStamp')
  Terminator : Terminator
  Terminator1 : Terminator
  TM_St : Outport
  tag scope: Agl_StSunEarth=global
  wires:
  Qib/1 -> StAMathModel/1(Qib), StAMathModel1/1(Qib), StAMathModel3/1(Qib), StAMathModel2/1(Qib)
  TC_St/1 -> StAMathModel/4(TC_St), StAMathModel1/4(TC_St), StAMathModel3/4(TC_St), StAMathModel2/4(TC_St)
  Mux/1 -> TM_St/1
  Constant10/1 -> StAMathModel2/3(Qsb_StAFix)
  Constant9/1 -> StAMathModel1/3(Qsb_StAFix)
  Constant11/1 -> StAMathModel3/3(Qsb_StAFix)
  Constant/1 -> StAMathModel/3(Qsb_StAFix)
  UTC_1970/1 -> Subsystem/1(UTC_1970)
  Subsystem/1(St_Time) -> Mux/7, Mux/5, Mux/3, Mux/1
  StAMathModel/1(TM_Data_StA) -> Mux/2
  StAMathModel1/1(TM_Data_StA) -> Mux/4
  StAMathModel2/1(TM_Data_StA) -> Mux/6
  StAMathModel3/1(TM_Data_StA) -> Mux/8
  StANoise/1 -> StAMathModel/2(Cons_StNoise)
  StBNoise/1 -> StAMathModel1/2(Cons_StNoise)
  StCNoise/1 -> StAMathModel2/2(Cons_StNoise)
  StDNoise/1 -> StAMathModel3/2(Cons_StNoise)
  Constant1/1 -> StAMathModel/5(StNum)
  Constant2/1 -> StAMathModel1/5(StNum)
  Constant3/1 -> StAMathModel2/5(StNum)
  Constant4/1 -> StAMathModel3/5(StNum)
  Constant5/1 -> Selector1/1, Selector7/1, Selector5/1, Selector4/1
  Constant6/1 -> Selector8/1, Selector6/1, Selector3/1, Selector2/1
  Qob/1 -> StAMathModel/10(Qob), StAMathModel1/10(Qob), StAMathModel3/10(Qob), StAMathModel2/10(Qob)
  Sun_b/1 -> StAMathModel/6(Sun_b), StAMathModel1/6(Sun_b), StAMathModel3/6(Sun_b), StAMathModel2/6(Sun_b)
  Sunshine/1 -> StAMathModel/7(Sunshine), StAMathModel1/7(Sunshine), StAMathModel3/7(Sunshine), StAMathModel2/7(Sunshine)
  Selector1/1 -> StAMathModel/8(SEA)
  Selector2/1 -> StAMathModel/9(EEA)
  Selector3/1 -> StAMathModel1/9(EEA)
  Selector4/1 -> StAMathModel1/8(SEA)
  Selector5/1 -> StAMathModel2/8(SEA)
  Selector6/1 -> StAMathModel2/9(EEA)
  Selector7/1 -> StAMathModel3/8(SEA)
  Selector8/1 -> StAMathModel3/9(EEA)
  StAMathModel2/2(Agl_St&SunEarth) -> Terminator/1
  StAMathModel3/2(Agl_St&SunEarth) -> Terminator1/1
  StAMathModel/2(Agl_St&SunEarth) -> Mux1/1
  StAMathModel1/2(Agl_St&SunEarth) -> Mux1/2
  Mux1/1 -> [Agl_StSunEarth]

== system GS_model/Subsystem2/Tc/GNSS1/Enabled Subsystem ==
  In1 : Inport
  Enable : EnablePort
  Data Store Write2 : DataStoreWrite  DataStoreName=Dyn_GNSS_PropagationTime1
  wires:
  In1/1 -> Data Store Write2/1

== system GS_model/Subsystem2/Tc/GNSS1/Enabled Subsystem1 ==
  In1 : Inport
  Enable : EnablePort
  Data Store Write2 : DataStoreWrite  DataStoreName=Dyn_GNSS_PropagationTime2
  wires:
  In1/1 -> Data Store Write2/1

== system GS_model/Subsystem2/Tc/Panel/double→8lowbit ==
  In1 : Inport
  Bitwise Operator : simulink/Logic and Bit Operations/Bitwise Operator  logicop=AND  UseBitMask=on  BitMask=bin2dec('00000001')  BitMaskRealWorld=Stored Integer
  Bitwise Operator1 : simulink/Logic and Bit Operations/Bitwise Operator  logicop=AND  UseBitMask=on  BitMask=bin2dec('00000010')  BitMaskRealWorld=Stored Integer
  Bitwise Operator2 : simulink/Logic and Bit Operations/Bitwise Operator  logicop=AND  UseBitMask=on  BitMask=bin2dec('00000100')  BitMaskRealWorld=Stored Integer
  Bitwise Operator3 : simulink/Logic and Bit Operations/Bitwise Operator  logicop=AND  UseBitMask=on  BitMask=bin2dec('00001000')  BitMaskRealWorld=Stored Integer
  Bitwise Operator4 : simulink/Logic and Bit Operations/Bitwise Operator  logicop=AND  UseBitMask=on  BitMask=bin2dec('00010000')  BitMaskRealWorld=Stored Integer
  Bitwise Operator5 : simulink/Logic and Bit Operations/Bitwise Operator  logicop=AND  UseBitMask=on  BitMask=bin2dec('00100000')  BitMaskRealWorld=Stored Integer
  Bitwise Operator6 : simulink/Logic and Bit Operations/Bitwise Operator  logicop=AND  UseBitMask=on  BitMask=bin2dec('01000000')  BitMaskRealWorld=Stored Integer
  Bitwise Operator7 : simulink/Logic and Bit Operations/Bitwise Operator  logicop=AND  UseBitMask=on  BitMask=bin2dec('10000000')  BitMaskRealWorld=Stored Integer
  Compare To Zero{,1..7} (8 alike) : simulink/Logic and Bit Operations/Compare To Zero  relop=>  OutDataTypeStr=boolean
  Data Type Conversion : DataTypeConversion  OutDataTypeStr=uint8
  Mux : Mux  Inputs=8
  Out1 : Outport
  wires:
  Data Type Conversion/1 -> Bitwise Operator7/1, Bitwise Operator6/1, Bitwise Operator5/1, Bitwise Operator4/1, Bitwise Operator3/1, Bitwise Operator2/1, Bitwise Operator1/1, Bitwise Operator/1
  Bitwise Operator1/1 -> Compare To Zero1/1
  Compare To Zero1/1 -> Mux/2
  Compare To Zero/1 -> Mux/1
  Bitwise Operator/1 -> Compare To Zero/1
  In1/1 -> Data Type Conversion/1
  Mux/1 -> Out1/1
  Bitwise Operator2/1 -> Compare To Zero2/1
  Bitwise Operator3/1 -> Compare To Zero3/1
  Bitwise Operator4/1 -> Compare To Zero4/1
  Bitwise Operator5/1 -> Compare To Zero5/1
  Bitwise Operator6/1 -> Compare To Zero6/1
  Bitwise Operator7/1 -> Compare To Zero7/1
  Compare To Zero2/1 -> Mux/3
  Compare To Zero3/1 -> Mux/4
  Compare To Zero4/1 -> Mux/5
  Compare To Zero5/1 -> Mux/6
  Compare To Zero6/1 -> Mux/7
  Compare To Zero7/1 -> Mux/8

== system GS_model/Subsystem2/Tc/Panel/double→8lowbit1 ==
  In1 : Inport
  Bitwise Operator : simulink/Logic and Bit Operations/Bitwise Operator  logicop=AND  UseBitMask=on  BitMask=bin2dec('00000001')  BitMaskRealWorld=Stored Integer
  Bitwise Operator1 : simulink/Logic and Bit Operations/Bitwise Operator  logicop=AND  UseBitMask=on  BitMask=bin2dec('00000010')  BitMaskRealWorld=Stored Integer
  Bitwise Operator2 : simulink/Logic and Bit Operations/Bitwise Operator  logicop=AND  UseBitMask=on  BitMask=bin2dec('00000100')  BitMaskRealWorld=Stored Integer
  Bitwise Operator3 : simulink/Logic and Bit Operations/Bitwise Operator  logicop=AND  UseBitMask=on  BitMask=bin2dec('00001000')  BitMaskRealWorld=Stored Integer
  Bitwise Operator4 : simulink/Logic and Bit Operations/Bitwise Operator  logicop=AND  UseBitMask=on  BitMask=bin2dec('00010000')  BitMaskRealWorld=Stored Integer
  Bitwise Operator5 : simulink/Logic and Bit Operations/Bitwise Operator  logicop=AND  UseBitMask=on  BitMask=bin2dec('00100000')  BitMaskRealWorld=Stored Integer
  Bitwise Operator6 : simulink/Logic and Bit Operations/Bitwise Operator  logicop=AND  UseBitMask=on  BitMask=bin2dec('01000000')  BitMaskRealWorld=Stored Integer
  Bitwise Operator7 : simulink/Logic and Bit Operations/Bitwise Operator  logicop=AND  UseBitMask=on  BitMask=bin2dec('10000000')  BitMaskRealWorld=Stored Integer
  Compare To Zero{,1..7} (8 alike) : simulink/Logic and Bit Operations/Compare To Zero  relop=>  OutDataTypeStr=boolean
  Data Type Conversion : DataTypeConversion  OutDataTypeStr=uint8
  Mux : Mux  Inputs=8
  Out1 : Outport
  wires:
  Compare To Zero7/1 -> Mux/8
  Compare To Zero6/1 -> Mux/7
  Compare To Zero5/1 -> Mux/6
  Compare To Zero4/1 -> Mux/5
  Compare To Zero3/1 -> Mux/4
  Compare To Zero2/1 -> Mux/3
  Bitwise Operator7/1 -> Compare To Zero7/1
  Bitwise Operator6/1 -> Compare To Zero6/1
  Bitwise Operator5/1 -> Compare To Zero5/1
  Bitwise Operator4/1 -> Compare To Zero4/1
  Bitwise Operator3/1 -> Compare To Zero3/1
  Bitwise Operator2/1 -> Compare To Zero2/1
  Mux/1 -> Out1/1
  In1/1 -> Data Type Conversion/1
  Bitwise Operator/1 -> Compare To Zero/1
  Compare To Zero/1 -> Mux/1
  Compare To Zero1/1 -> Mux/2
  Bitwise Operator1/1 -> Compare To Zero1/1
  Data Type Conversion/1 -> Bitwise Operator/1, Bitwise Operator1/1, Bitwise Operator2/1, Bitwise Operator3/1, Bitwise Operator4/1, Bitwise Operator5/1, Bitwise Operator6/1, Bitwise Operator7/1

== system GS_model/Subsystem2/Tc/QV2/double→4lowbit ==
  In1 : Inport
  Bitwise Operator : simulink/Logic and Bit Operations/Bitwise Operator  logicop=AND  UseBitMask=on  BitMask=bin2dec('00000001')  BitMaskRealWorld=Stored Integer
  Bitwise Operator1 : simulink/Logic and Bit Operations/Bitwise Operator  logicop=AND  UseBitMask=on  BitMask=bin2dec('00000010')  BitMaskRealWorld=Stored Integer
  Bitwise Operator2 : simulink/Logic and Bit Operations/Bitwise Operator  logicop=AND  UseBitMask=on  BitMask=bin2dec('00000100')  BitMaskRealWorld=Stored Integer
  Bitwise Operator3 : simulink/Logic and Bit Operations/Bitwise Operator  logicop=AND  UseBitMask=on  BitMask=bin2dec('00001000')  BitMaskRealWorld=Stored Integer
  Compare To Zero{,1..3} (4 alike) : simulink/Logic and Bit Operations/Compare To Zero  relop=>  OutDataTypeStr=boolean
  Data Type Conversion : DataTypeConversion  OutDataTypeStr=uint8
  Mux : Mux
  Out1 : Outport
  wires:
  Data Type Conversion/1 -> Bitwise Operator2/1, Bitwise Operator3/1, Bitwise Operator1/1, Bitwise Operator/1
  Bitwise Operator1/1 -> Compare To Zero1/1
  Compare To Zero1/1 -> Mux/2
  Compare To Zero/1 -> Mux/1
  Bitwise Operator/1 -> Compare To Zero/1
  In1/1 -> Data Type Conversion/1
  Mux/1 -> Out1/1
  Bitwise Operator2/1 -> Compare To Zero2/1
  Bitwise Operator3/1 -> Compare To Zero3/1
  Compare To Zero2/1 -> Mux/3
  Compare To Zero3/1 -> Mux/4

== system GS_model/Subsystem2/Tc/Reset1/Subsystem3 ==
  note: '11'--轨道闭环，姿态开环
      | ‘22’--轨道、姿态均闭环
      | ‘33’--轨道、姿态均开环
      | '11/22/33'均更新初值
  "command_word " : Inport
  Data Type Conversion : DataTypeConversion  OutDataTypeStr=double
  Data Type Conversion1 : DataTypeConversion  OutDataTypeStr=double
  Detect Rise Positive1 : simulink/Logic and Bit Operations/Detect Rise Positive  vinit=0  OutDataTypeStr=boolean
  Detect Rise Positive2 : simulink/Logic and Bit Operations/Detect Rise Positive  vinit=0  OutDataTypeStr=boolean
  Hex '11' : simulink/Logic and Bit Operations/Compare To Constant  relop===  const=17  OutDataTypeStr=boolean
  Hex '22' : simulink/Logic and Bit Operations/Compare To Constant  relop===  const=34  OutDataTypeStr=boolean
  Hex '33' : simulink/Logic and Bit Operations/Compare To Constant  relop===  const=51  OutDataTypeStr=boolean
  Logical Operator : Logic  Operator=OR  Inputs=3  AllPortsSameDT=off  OutDataTypeStr=boolean
  Logical Operator1 : Logic  Operator=OR  Inputs=3  AllPortsSameDT=off  OutDataTypeStr=boolean
  OrbitReset : Outport
  AttReset : Outport  Port=2
  wires:
  Logical Operator/1 -> Data Type Conversion1/1
  Hex '22'/1 -> Detect Rise Positive1/1
  "command_word "/1 -> Hex '33'/1, Hex '22'/1, Hex '11'/1
  Hex '11'/1 -> Detect Rise Positive2/1, Logical Operator/3
  Detect Rise Positive2/1 -> Logical Operator1/1
  Detect Rise Positive1/1 -> Logical Operator/2, Logical Operator1/2
  Hex '33'/1 -> Logical Operator/1, Logical Operator1/3
  Logical Operator1/1 -> Data Type Conversion/1
  Data Type Conversion/1 -> OrbitReset/1
  Data Type Conversion1/1 -> AttReset/1

== system GS_model/Subsystem2/Tc/SADA2/double→4lowbit ==
  In1 : Inport
  Bitwise Operator : simulink/Logic and Bit Operations/Bitwise Operator  logicop=AND  UseBitMask=on  BitMask=bin2dec('00000001')  BitMaskRealWorld=Stored Integer
  Bitwise Operator1 : simulink/Logic and Bit Operations/Bitwise Operator  logicop=AND  UseBitMask=on  BitMask=bin2dec('00000010')  BitMaskRealWorld=Stored Integer
  Bitwise Operator2 : simulink/Logic and Bit Operations/Bitwise Operator  logicop=AND  UseBitMask=on  BitMask=bin2dec('00000100')  BitMaskRealWorld=Stored Integer
  Bitwise Operator3 : simulink/Logic and Bit Operations/Bitwise Operator  logicop=AND  UseBitMask=on  BitMask=bin2dec('00001000')  BitMaskRealWorld=Stored Integer
  Bitwise Operator4 : simulink/Logic and Bit Operations/Bitwise Operator  logicop=AND  UseBitMask=on  BitMask=bin2dec('00010000')  BitMaskRealWorld=Stored Integer
  Bitwise Operator5 : simulink/Logic and Bit Operations/Bitwise Operator  logicop=AND  UseBitMask=on  BitMask=bin2dec('00100000')  BitMaskRealWorld=Stored Integer
  Compare To Zero{,1..5} (6 alike) : simulink/Logic and Bit Operations/Compare To Zero  relop=>  OutDataTypeStr=boolean
  Data Type Conversion : DataTypeConversion  OutDataTypeStr=uint8
  Mux : Mux  Inputs=6
  Out1 : Outport
  wires:
  Data Type Conversion/1 -> Bitwise Operator2/1, Bitwise Operator5/1, Bitwise Operator4/1, Bitwise Operator3/1, Bitwise Operator1/1, Bitwise Operator/1
  Bitwise Operator1/1 -> Compare To Zero1/1
  Compare To Zero1/1 -> Mux/2
  Compare To Zero/1 -> Mux/1
  Bitwise Operator/1 -> Compare To Zero/1
  In1/1 -> Data Type Conversion/1
  Mux/1 -> Out1/1
  Bitwise Operator2/1 -> Compare To Zero2/1
  Bitwise Operator3/1 -> Compare To Zero3/1
  Compare To Zero2/1 -> Mux/3
  Compare To Zero3/1 -> Mux/4
  Bitwise Operator4/1 -> Compare To Zero4/1
  Bitwise Operator5/1 -> Compare To Zero5/1
  Compare To Zero4/1 -> Mux/5
  Compare To Zero5/1 -> Mux/6

== system GS_model/Subsystem2/Tc/Time1/YMDHMS 2 S ==
  note: 1
  note: Y
  note: M
  note: 3
  note: 1
  note: D
  note: 1
  YMDHMS : Inport
  Constant1 : Constant  Value=UTC_0to1970
  Demux1 : Demux  Outputs=[1 1 3 1]
  Display : Display
  Display1 : Display
  Gain : Gain  Gain=K_Day2Sec
  Mux1 : Mux  Inputs=[3,1]
  Mux2 : Mux  Inputs=3
  Subsystem1 : Subsystem
  Sum1 : Sum  Inputs=|+-  SaturateOnIntegerOverflow=on
  days8 : Fcn  Expr=u(1)+(u(2)+u(3)/60+u(4)/3600)/24
  UTC_1970 : Outport
  wires:
  Demux1/1 -> Mux2/1
  Mux2/1 -> Subsystem1/1(In)
  Constant1/1 -> Sum1/2
  Mux1/1 -> days8/1
  Demux1/4 -> Mux1/2
  Demux1/2 -> Mux2/2
  days8/1 -> Mux2/3
  Demux1/3 -> Mux1/1
  Subsystem1/1(Out) -> Gain/1
  YMDHMS/1 -> Display1/1, Demux1/1
  Gain/1 -> Sum1/1
  Sum1/1 -> Display/1, UTC_1970/1

== system GS_model/Subsystem2/EquipmentCmd/Fw1/Subsystem7/Subsystem1 ==
  note: 1 -- FW_Spd_422
      | 2 -- FW_Spd_UDP
      | 3 -- FW_Spd_FC
      |
      | 4 -- FW_T_422
      | 5 -- FW_T_UDP
      | 6 -- FW_T_FC
      |
      | 7 -- FW_Mode_422
      | 8 -- FW_Mode_UDP
      | 9 -- FW_Mode_FC
      |
      | 10--FW_DataSource
  note: FW_DataSource
      | AA-真采集（默认）  1-422(DB9);
      |                                  0-反测（默认
      | 55 -伪采集                UDP
  FWNum : Inport
  FW_Cmd : Inport  Port=2
  TC_Fw : Inport  Port=3
  Compare To Constant : simulink/Logic and Bit Operations/Compare To Constant  relop===  const=0  OutDataTypeStr=boolean
  Demux : Demux  Outputs=[9;1]
  Demux2 : Demux  Outputs=[1;2]
  FWDataSourceChoice : Subsystem
      mask Display: disp('FWDataSourceChoice')
  Logical Operator : Logic  Operator=OR  AllPortsSameDT=off  OutDataTypeStr=boolean
  Mux : Mux  Inputs=3
  Mux1 : Mux  Inputs=2
  Relational Operator1 : RelationalOperator  Operator===  OutDataTypeStr=boolean  RndMeth=Simplest
  Selector : Selector  InputPortWidth=3  IndexOptions=Index vector (dialog)  Indices=[2 3 1]  OutputSizes=1
  Selector2 : Selector  InputPortWidth=23  IndexOptions=Index vector (dialog)  Indices=[1 2]  OutputSizes=1
  Triggered Subsystem1 : Subsystem  TreatAsAtomicUnit=on
      mask Display: disp('FWChoice')
  Cmd_Mode/Spd/T : Outport
  wires:
  Mux/1 -> Cmd_Mode/Spd/T/1
  FWDataSourceChoice/1(Cmd_Mode) -> Mux/1
  Demux/1 -> FWDataSourceChoice/2(FW_Cmd)
  Demux/2 -> Mux1/1
  FW_Cmd/1 -> Demux/1
  TC_Fw/1 -> Selector2/1
  Selector2/1 -> Mux1/2
  FWDataSourceChoice/3(Cmd_T) -> Mux/3
  FWDataSourceChoice/2(Cmd_Spd) -> Mux/2
  Compare To Constant/1 -> Logical Operator/2
  Triggered Subsystem1/1(Out1) -> FWDataSourceChoice/1(FW_Data_Source)
  Mux1/1 -> Selector/1
  Demux2/2 -> Triggered Subsystem1/1(In1)
  Selector/1 -> Demux2/1
  Relational Operator1/1 -> Logical Operator/1
  Logical Operator/1 -> Triggered Subsystem1/Enable
  Demux2/1 -> Compare To Constant/1, Relational Operator1/2
  FWNum/1 -> Relational Operator1/1

== system GS_model/Subsystem2/EquipmentCmd/Fw1/Subsystem7/Subsystem2 ==
  note: FW_DataSource
      | AA-真采集（默认）  1-422(DB9);
      |                                  0-反测（默认
      | 55 -伪采集                UDP
  note: 1 -- FW_Spd_422
      | 2 -- FW_Spd_UDP
      | 3 -- FW_Spd_FC
      |
      | 4 -- FW_T_422
      | 5 -- FW_T_UDP
      | 6 -- FW_T_FC
      |
      | 7 -- FW_Mode_422
      | 8 -- FW_Mode_UDP
      | 9 -- FW_Mode_FC
      |
      | 10--FW_DataSource
  FWNum : Inport
  FW_Cmd : Inport  Port=2
  TC_Fw : Inport  Port=3
  Compare To Constant : simulink/Logic and Bit Operations/Compare To Constant  relop===  const=0  OutDataTypeStr=boolean
  Demux : Demux  Outputs=[9;1]
  Demux2 : Demux  Outputs=[1;2]
  FWDataSourceChoice : Subsystem
      mask Display: disp('FWDataSourceChoice')
  Logical Operator : Logic  Operator=OR  AllPortsSameDT=off  OutDataTypeStr=boolean
  Mux : Mux  Inputs=3
  Mux1 : Mux  Inputs=2
  Relational Operator1 : RelationalOperator  Operator===  OutDataTypeStr=boolean  RndMeth=Simplest
  Selector : Selector  InputPortWidth=3  IndexOptions=Index vector (dialog)  Indices=[2 3 1]  OutputSizes=1
  Selector2 : Selector  InputPortWidth=23  IndexOptions=Index vector (dialog)  Indices=[1 2]  OutputSizes=1
  Triggered Subsystem1 : Subsystem  TreatAsAtomicUnit=on
      mask Display: disp('FWChoice')
  Cmd_Mode/Spd/T : Outport
  wires:
  FWNum/1 -> Relational Operator1/1
  Demux2/1 -> Relational Operator1/2, Compare To Constant/1
  Logical Operator/1 -> Triggered Subsystem1/Enable
  Relational Operator1/1 -> Logical Operator/1
  Selector/1 -> Demux2/1
  Demux2/2 -> Triggered Subsystem1/1(In1)
  Mux1/1 -> Selector/1
  Triggered Subsystem1/1(Out1) -> FWDataSourceChoice/1(FW_Data_Source)
  Compare To Constant/1 -> Logical Operator/2
  FWDataSourceChoice/2(Cmd_Spd) -> Mux/2
  FWDataSourceChoice/3(Cmd_T) -> Mux/3
  Selector2/1 -> Mux1/2
  TC_Fw/1 -> Selector2/1
  FW_Cmd/1 -> Demux/1
  Demux/2 -> Mux1/1
  Demux/1 -> FWDataSourceChoice/2(FW_Cmd)
  FWDataSourceChoice/1(Cmd_Mode) -> Mux/1
  Mux/1 -> Cmd_Mode/Spd/T/1
